simulink model "plant_block"  (R2019b)
settings: Solver=ode1  StartTime=0.0  StopTime=300  RelTol=1e-3  EnableMultiTasking=on
undefined symbols (not defined in the file or in its folder): K4
libraries: simulink x2
settings Model: SimulationMode=external  Creator=Dro  LastModifiedBy=s4581164
settings DataIOCC: LimitDataPoints=on  SaveFormat=Array  SignalLoggingSaveFormat=ModelDataLogs  ReturnWorkspaceOutputs=off  SignalLoggingName=sigsOut
settings OptimizationCC: ExpressionDepthLimit=2147483647  InitFltsAndDblsToZero=on
settings DebuggingCC: SaveWithParameterizedLinksMsg=none  UnderspecifiedInitializationDetection=Classic  MergeDetectMultiDrivingBlocksExec=none  SignalResolutionControl=TryResolveAllWithWarning  MultiTaskDSMMsg=warning  MultiTaskCondExecSysMsg=none  FcnCallInpInsideContextMsg=warning  StateNameClashWarn=warning  SFUnexpectedBacktrackingDiag=warning  SFNoUnconditionalDefaultTransitionDiag=warning  SFExecutionAtInitializationDiag=none  ArithmeticOperatorsInVariantConditions=warning
settings HardwareCC: TargetBitPerLong=64  TargetBitPerPointer=64  TargetIntDivRoundTo=Zero  TargetEndianess=LittleEndian  TargetWordSize=64  TargetHWDeviceType=Intel->x86-64
settings ModelReferenceCC: PropagateSignalLabelsOutOfModel=off
settings SFSimCC: SimUseLocalCustomCode=off  CustomCodeUndefinedFunction=UseInterfaceOnly
settings RTWCC: Description=Simulink Desktop Real-Time  SystemTargetFile=sldrt.tlc  TemplateMakefile=sldrt.tmf  RTWUseLocalCustomCode=off  RTWCompilerOptimization=on
settings CodeAppCC: MaxIdLength=95  StateflowObjectComments=on
settings TargetCC: TargetPreCompLibLocation=C:\Program Files\MATLAB\R2019b\toolbox\sldrt\lib\win64  ModelReferenceCompliant=off  CompOptLevelCompliant=off  GeneratePreprocessorConditionals=Use local settings  PreserveStateflowLocalDataDimensions=off
settings ConfigComp: CovMetricSettings=dw  CovHtmlReporting=on  CovSaveCumulativeToWorkspaceVar=on  CovSaveSingleToWorkspaceVar=on  CovExternalEMLEnable=off

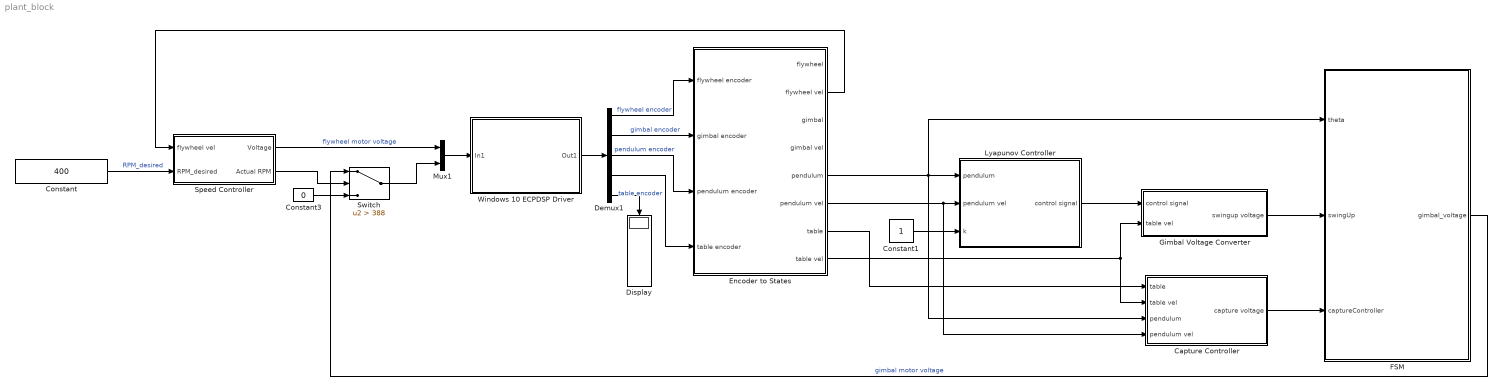
== system plant_block ==
  Capture Controller : Subsystem
  Constant : Constant  Value=400
  Constant1 : Constant
  Constant3 : Constant  Value=0
  Demux1 : Demux  Outputs=5
  Display : Display
  Encoder to States : Subsystem
  FSM : Stateflow chart  BlockKeywords=__PRM__SERIALIZED__DATA__:Stateflow Chart,Stateflow Diagram  TreatAsAtomicUnit=on
  Gimbal Voltage Converter : Subsystem
  Lyapunov Controller : Subsystem
  Mux1 : Mux  Inputs=2
  "Speed Controller " : Subsystem
  Switch : Switch  Criteria=u2 > Threshold  Threshold=388
  Windows 10 ECPDSP Driver : Subsystem  mask{BaseAddr='0xD000', STime=0.008, TimeOutPer=500, HWAccess=on}
      mask prompts: BaseAddr "Base I/O Address"; STime "Sample Time (Sec)"; TimeOutPer "Timeout Period (500 ~ 2000)"; HWAccess "Hardware Access"
      mask Display: color('black');disp('ECPDSP Driver\n upto\n 4 Encs(ADC Channels)\n and 2 Dacs')
  wires:
  Mux1/1 -> Windows 10 ECPDSP Driver/1(In1)
  "Speed Controller "/1(Voltage) -> Mux1/1  "flywheel motor voltage"
  Demux1/1 -> Encoder to States/1(flywheel encoder)  "flywheel encoder"
  Demux1/2 -> Encoder to States/2(gimbal encoder)  "gimbal encoder"
  Demux1/3 -> Encoder to States/3(pendulum encoder)  "pendulum encoder"
  Demux1/4 -> Encoder to States/4(table encoder)  "table encoder"
  FSM/1(gimbal_voltage) -> Switch/1  "gimbal motor voltage"
  Windows 10 ECPDSP Driver/1(Out1) -> Demux1/1
  Constant/1 -> "Speed Controller "/2(RPM_desired)  "RPM_desired"
  Encoder to States/6(pendulum vel) -> Capture Controller/4(pendulum vel), Lyapunov Controller/2(pendulum vel)
  Constant1/1 -> Lyapunov Controller/3(k)
  Encoder to States/2(flywheel vel) -> "Speed Controller "/1(flywheel vel)
  Lyapunov Controller/1(control signal) -> Gimbal Voltage Converter/1(control signal)
  Encoder to States/8(table vel) -> Capture Controller/2(table vel), Gimbal Voltage Converter/2(table vel)
  Encoder to States/5(pendulum) -> FSM/1(theta), Lyapunov Controller/1(pendulum), Capture Controller/3(pendulum)
  Gimbal Voltage Converter/1(swingup voltage) -> FSM/2(swingUp)
  Capture Controller/1(capture voltage) -> FSM/3(captureController)
  Encoder to States/7(table) -> Capture Controller/1(table)
  Switch/1 -> Mux1/2
  "Speed Controller "/2("Actual RPM ") -> Switch/2
  Constant3/1 -> Switch/3
  Demux1/5 -> Display/1

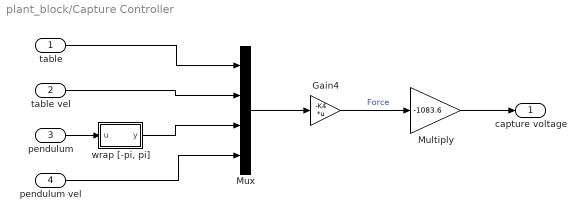
== system plant_block/Capture Controller ==
  table : Inport
  table vel : Inport  Port=2
  pendulum : Inport  Port=3
  pendulum vel : Inport  Port=4
  Gain4 : Gain  Gain=-K4  Multiplication=Matrix(K*u)
  Multiply : Gain  Gain=-1083.6
  Mux : Mux
  "wrap [-pi, pi]" : MATLAB Function  TreatAsAtomicUnit=on
  capture voltage : Outport
  wires:
  table/1 -> Mux/1
  table vel/1 -> Mux/2
  pendulum vel/1 -> Mux/4
  Mux/1 -> Gain4/1
  Multiply/1 -> capture voltage/1
  Gain4/1 -> Multiply/1  "Force"
  pendulum/1 -> "wrap [-pi, pi]"/1(u)
  "wrap [-pi, pi]"/1(y) -> Mux/3

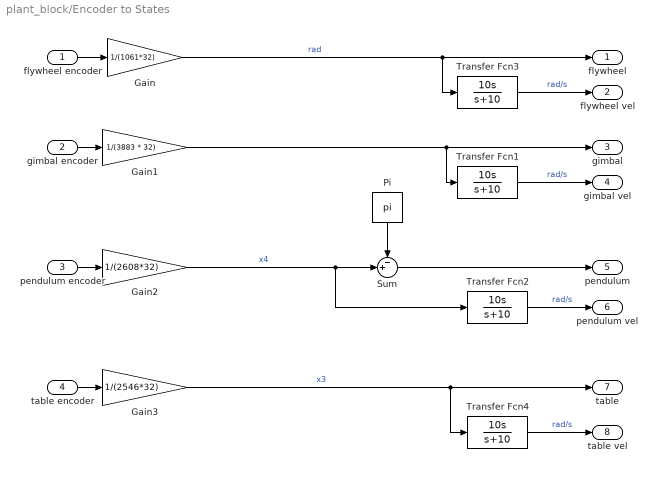
== system plant_block/Encoder to States ==
  flywheel encoder : Inport
  gimbal encoder : Inport  Port=2
  pendulum encoder : Inport  Port=3
  table encoder : Inport  Port=4
  Gain : Gain  Gain=1/(1061*32)
  Gain1 : Gain  Gain=1/(3883 * 32)
  Gain2 : Gain  Gain=1/(2608*32)
  Gain3 : Gain  Gain=1/(2546*32)
  Pi : Constant  Value=pi  OutDataTypeStr=Inherit: Inherit via back propagation
  Sum : Sum  Inputs=-+|
  Transfer Fcn{1..4} (4 alike) : TransferFcn  Numerator=[10 0 ]  Denominator=[1 10]
  flywheel : Outport
  flywheel vel : Outport  Port=2
  gimbal : Outport  Port=3
  gimbal vel : Outport  Port=4
  pendulum : Outport  Port=5
  pendulum vel : Outport  Port=6
  table : Outport  Port=7
  table vel : Outport  Port=8
  wires:
  flywheel encoder/1 -> Gain/1
  gimbal encoder/1 -> Gain1/1
  pendulum encoder/1 -> Gain2/1
  table encoder/1 -> Gain3/1
  Gain/1 -> Transfer Fcn3/1, flywheel/1  "rad"
  Transfer Fcn3/1 -> flywheel vel/1  "rad/s"
  Gain1/1 -> Transfer Fcn1/1, gimbal/1
  Transfer Fcn1/1 -> gimbal vel/1  "rad/s"
  Transfer Fcn2/1 -> pendulum vel/1  "rad/s"
  Gain3/1 -> Transfer Fcn4/1, table/1  "x3"
  Transfer Fcn4/1 -> table vel/1  "rad/s"
  Sum/1 -> pendulum/1
  Pi/1 -> Sum/1
  Gain2/1 -> Transfer Fcn2/1, Sum/2  "x4"

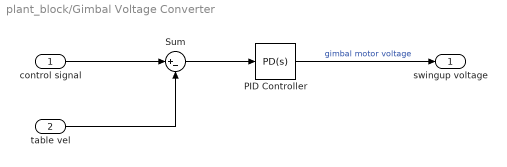
== system plant_block/Gimbal Voltage Converter ==
  control signal : Inport
  table vel : Inport  Port=2
  PID Controller : simulink/Continuous/PID Controller  Controller=PD  Form=Parallel  TimeDomain=Continuous-time  SampleTime=-1  IntegratorMethod=Forward Euler  FilterMethod=Forward Euler  ControllerParametersSource=internal  P=3870  I=0  D=0  UseFilter=on  N=100  TunerSelectOption=Transfer Function Based (PID Tuner App)  InitialConditionSource=internal  InitialConditionForIntegrator=0  InitialConditionForFilter=0  DifferentiatorICPrevScaledInput=0  ExternalReset=none  TrackingMode=off  Kt=1  LimitOutput=off  UpperSaturationLimit=inf  LowerSaturationLimit=-inf  LinearizeAsGain=on  AntiWindupMode=none  Kb=1  POutMin=[]  POutMax=[]  IOutMin=[]  IOutMax=[]  DOutMin=[]  DOutMax=[]  NOutMin=[]  NOutMax=[]  SumOutMin=[]  SumOutMax=[]  SaturationOutMin=[]  SaturationOutMax=[]  PParamMin=[]  PParamMax=[]  IParamMin=[]  IParamMax=[]  DParamMin=[]  DParamMax=[]  NParamMin=[]  NParamMax=[]  KbParamMin=[]  KbParamMax=[]  KtParamMin=[]  KtParamMax=[]  KbOutMin=[]  KbOutMax=[]  KtOutMin=[]  KtOutMax=[]  IntegratorOutMin=[]  IntegratorOutMax=[]  FilterOutMin=[]  FilterOutMax=[]  SumI1OutMin=[]  SumI1OutMax=[]  SumI2OutMin=[]  SumI2OutMax=[]  SumI3OutMin=[]  SumI3OutMax=[]  SumI4OutMin=[]  SumI4OutMax=[]  SumDOutMin=[]  SumDOutMax=[]  DifferentiatorOutMin=[]  DifferentiatorOutMax=[]  FilterDiffOutCoefMin=[]  FilterDiffOutCoefMax=[]  ReciprocalOutMin=[]  ReciprocalOutMax=[]  SumDenOutMin=[]  SumDenOutMax=[]  SumNumOutMin=[]  SumNumOutMax=[]  DivideOutMin=[]  DivideOutMax=[]  IntegratorContinuousStateAttributes=''  IntegratorStateMustResolveToSignalObject=off  IntegratorRTWStateStorageClass=Auto  FilterContinuousStateAttributes=''  FilterStateMustResolveToSignalObject=off  FilterRTWStateStorageClass=Auto  ParallelPVariant=InternalParameters  IdealPVariant=Disabled  IVariant=Disabled  DVariant=InternalParameters  IntegratorVariant=Disabled  SatVariant=Disabled  AWVariant=Disabled  PCopyVariant=Disabled  TRVariant=Disabled  FdbkBlocksVariant=Forward  IdealPFdbkVariant=Disabled  SatFdbkVariant=Disabled  DerivativeFilterVariant=ContFilter  NVariant=InternalParameters  NCopyVariant=Disabled  FilterICVariant=InternalICsFilter  IntegratorICVariant=Disabled  ExternalResetVariant=Disabled  TRSumVariant=Passthrough  SumFdbkVariant=Disabled  SumVariant=Sum_PD
  Sum : Sum  Inputs=|+-
  swingup voltage : Outport
  wires:
  PID Controller/1 -> swingup voltage/1  "gimbal motor voltage"
  control signal/1 -> Sum/1
  table vel/1 -> Sum/2
  Sum/1 -> PID Controller/1

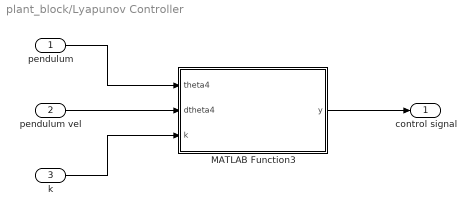
== system plant_block/Lyapunov Controller ==
  pendulum : Inport
  pendulum vel : Inport  Port=2
  k : Inport  Port=3
  MATLAB Function3 : MATLAB Function  TreatAsAtomicUnit=on
  control signal : Outport
  wires:
  k/1 -> MATLAB Function3/3(k)
  pendulum vel/1 -> MATLAB Function3/2(dtheta4)
  pendulum/1 -> MATLAB Function3/1(theta4)
  MATLAB Function3/1(y) -> control signal/1

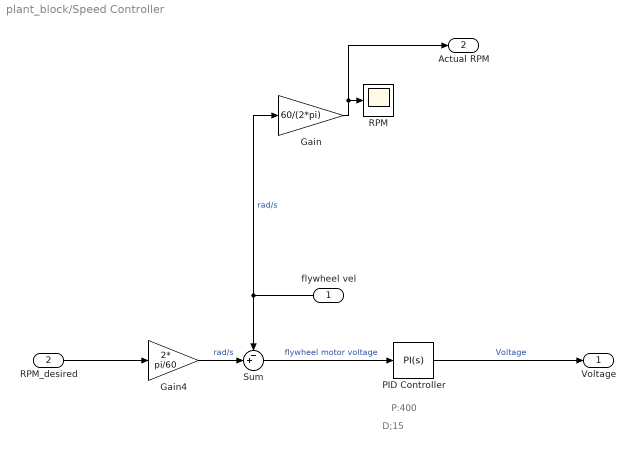
== system plant_block/Speed Controller  ==
  note: D;15
  note: P:400
  flywheel vel : Inport
  RPM_desired : Inport  Port=2
  Gain : Gain  Gain=60/(2*pi)
  Gain4 : Gain  Gain=2* pi/60
  PID Controller : simulink/Continuous/PID Controller  Controller=PI  Form=Parallel  TimeDomain=Continuous-time  SampleTime=-1  IntegratorMethod=Forward Euler  FilterMethod=Forward Euler  ControllerParametersSource=internal  P=400  I=15  D=0  UseFilter=on  N=100  TunerSelectOption=Transfer Function Based (PID Tuner App)  InitialConditionSource=internal  InitialConditionForIntegrator=0  InitialConditionForFilter=0  DifferentiatorICPrevScaledInput=0  ExternalReset=none  TrackingMode=off  Kt=1  LimitOutput=off  UpperSaturationLimit=inf  LowerSaturationLimit=-inf  LinearizeAsGain=on  AntiWindupMode=none  Kb=1  POutMin=[]  POutMax=[]  IOutMin=[]  IOutMax=[]  DOutMin=[]  DOutMax=[]  NOutMin=[]  NOutMax=[]  SumOutMin=[]  SumOutMax=[]  SaturationOutMin=[]  SaturationOutMax=[]  PParamMin=[]  PParamMax=[]  IParamMin=[]  IParamMax=[]  DParamMin=[]  DParamMax=[]  NParamMin=[]  NParamMax=[]  KbParamMin=[]  KbParamMax=[]  KtParamMin=[]  KtParamMax=[]  KbOutMin=[]  KbOutMax=[]  KtOutMin=[]  KtOutMax=[]  IntegratorOutMin=[]  IntegratorOutMax=[]  FilterOutMin=[]  FilterOutMax=[]  SumI1OutMin=[]  SumI1OutMax=[]  SumI2OutMin=[]  SumI2OutMax=[]  SumI3OutMin=[]  SumI3OutMax=[]  SumI4OutMin=[]  SumI4OutMax=[]  SumDOutMin=[]  SumDOutMax=[]  DifferentiatorOutMin=[]  DifferentiatorOutMax=[]  FilterDiffOutCoefMin=[]  FilterDiffOutCoefMax=[]  ReciprocalOutMin=[]  ReciprocalOutMax=[]  SumDenOutMin=[]  SumDenOutMax=[]  SumNumOutMin=[]  SumNumOutMax=[]  DivideOutMin=[]  DivideOutMax=[]  IntegratorContinuousStateAttributes=''  IntegratorStateMustResolveToSignalObject=off  IntegratorRTWStateStorageClass=Auto  FilterContinuousStateAttributes=''  FilterStateMustResolveToSignalObject=off  FilterRTWStateStorageClass=Auto  ParallelPVariant=InternalParameters  IdealPVariant=Disabled  IVariant=InternalParameters  DVariant=Disabled  IntegratorVariant=Continuous  SatVariant=Disabled  AWVariant=Passthrough  PCopyVariant=Disabled  TRVariant=Disabled  FdbkBlocksVariant=Forward  IdealPFdbkVariant=Disabled  SatFdbkVariant=Disabled  DerivativeFilterVariant=Disabled  NVariant=Disabled  NCopyVariant=Disabled_SignalSpec  FilterICVariant=Disabled  IntegratorICVariant=InternalICs  ExternalResetVariant=Disabled  TRSumVariant=Passthrough  SumFdbkVariant=Disabled  SumVariant=Sum_PI
  RPM : Scope
  Sum : Sum  Inputs=-+|
  Voltage : Outport
  "Actual RPM " : Outport  Port=2
  wires:
  Gain4/1 -> Sum/2  "rad/s"
  flywheel vel/1 -> Gain/1, Sum/1  "rad/s"
  Sum/1 -> PID Controller/1  "flywheel motor voltage"
  PID Controller/1 -> Voltage/1  "Voltage"
  RPM_desired/1 -> Gain4/1
  Gain/1 -> "Actual RPM "/1, RPM/1

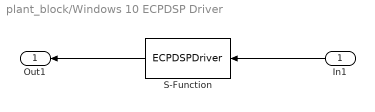
== system plant_block/Windows 10 ECPDSP Driver ==
  In1 : Inport
  S-Function : S-Function  FunctionName=ECPDSPDriver  Parameters=BaseAddr,STime,TimeOutPer,HWAccess  SFunctionDeploymentMode=off  EnableBusSupport=off
  Out1 : Outport
  wires:
  In1/1 -> S-Function/1
  S-Function/1 -> Out1/1

== matlab function plant_block/Capture Controller/wrap [-pi, pi] ==
  data: u input; y output
function y = fcn(u)
y = u - 2*pi*floor((u+pi)/(2*pi));
end

== stateflow chart plant_block/FSM ==
  state SwingUp
    entry:
    gimbal_voltage = swingUp
  state CaptureController
    entry:
    gimbal_voltage = captureController
  SwingUp -> CaptureController : [abs(theta) < 0.02]
  (default) -> SwingUp
  CaptureController -> SwingUp : [abs(theta) > 0.8]
  data: theta input; swingUp input; gimbal_voltage output; captureController input

== matlab function plant_block/Lyapunov Controller/MATLAB Function3 ==
  data: theta4 input; y output; dtheta4 input; k input
function y = fcn(theta4, dtheta4, k)
m = 0.1580;
lcg = 0.2698;
rh = 0.37;
J1 = 0.1314;
Jz_bar = 0.0131;
g = 9.81;
c = 0.002;
Eo = 0;
Id = 0.0148;
dtheta1 = 400 * (2*pi/60);

E = 0.5*m*lcg^2*dtheta4^2 + m*g*lcg*(cos(theta4) - 1);

y = -k *(E - Eo)*dtheta4*cos(theta4);
end
